simulink model "testCurrentPMSM"  (R2023a)
settings: Solver=ode15s  StartTime=0.0  StopTime=2.0  RelTol=1e-3
libraries: slpidlib x2, eePmsmFieldOrientedControl x1
settings Model: Creator=admin  LastModifiedBy=admin

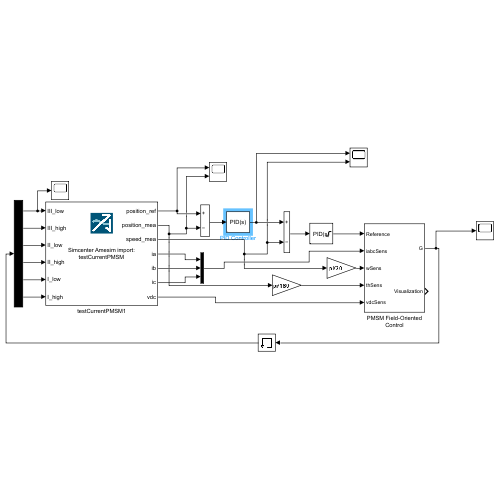
[thumbnail: Simulink's stored preview of the top-level diagram]
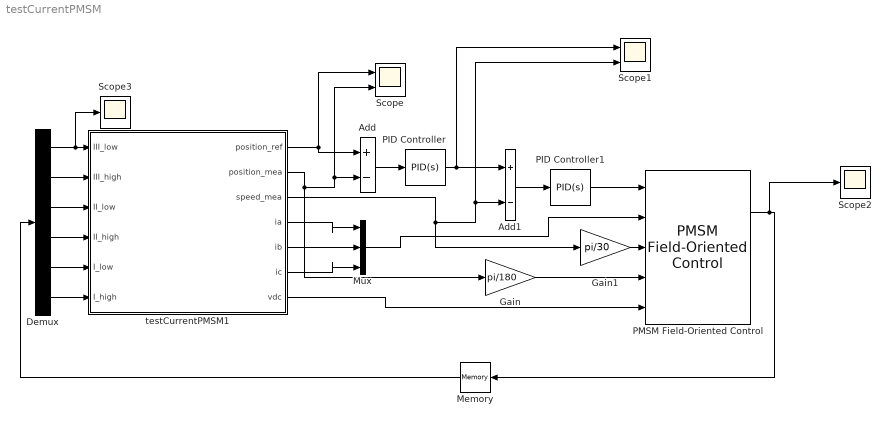
== system testCurrentPMSM ==
  Add : Sum  Inputs=+-
  Add1 : Sum  Inputs=+-
  Demux : Demux  Outputs=6
  Gain : Gain  Gain=pi/180
  Gain1 : Gain  Gain=pi/30
  Memory : Memory
  Mux : Mux  Inputs=3
  PID Controller : slpidlib/PID Controller  Controller=PID  Form=Parallel  TimeDomain=Continuous-time  UseExternalTs=off  SampleTime=-1  IntegratorMethod=Forward Euler  FilterMethod=Forward Euler  ControllerParametersSource=internal  P=1  I=0  UseKiTs=off  D=0  N=100  UseFilter=on  TunerSelectOption=Transfer Function Based (PID Tuner App)  InitialConditionSource=internal  InitialConditionForIntegrator=0  InitialConditionForFilter=0  DifferentiatorICPrevScaledInput=0  ExternalReset=none  TrackingMode=off  Kt=1  LimitOutput=off  SatLimitsSource=internal  UpperSaturationLimit=1000  LowerSaturationLimit=-1000  LinearizeAsGain=on  AntiWindupMode=none  Kb=1  LimitIntegrator=off  UpperIntegratorSaturationLimit=inf  LowerIntegratorSaturationLimit=-inf  POutMin=[]  POutMax=[]  IOutMin=[]  IOutMax=[]  DOutMin=[]  DOutMax=[]  NOutMin=[]  NOutMax=[]  SumOutMin=[]  SumOutMax=[]  SaturationOutMin=[]  SaturationOutMax=[]  PParamMin=[]  PParamMax=[]  IParamMin=[]  IParamMax=[]  DParamMin=[]  DParamMax=[]  NParamMin=[]  NParamMax=[]  KbParamMin=[]  KbParamMax=[]  KtParamMin=[]  KtParamMax=[]  KbOutMin=[]  KbOutMax=[]  KtOutMin=[]  KtOutMax=[]  IntegratorOutMin=[]  IntegratorOutMax=[]  FilterOutMin=[]  FilterOutMax=[]  SumI1OutMin=[]  SumI1OutMax=[]  SumI2OutMin=[]  SumI2OutMax=[]  SumI3OutMin=[]  SumI3OutMax=[]  SumI4OutMin=[]  SumI4OutMax=[]  SumDOutMin=[]  SumDOutMax=[]  DifferentiatorOutMin=[]  DifferentiatorOutMax=[]  FilterDiffOutCoefMin=[]  FilterDiffOutCoefMax=[]  ReciprocalOutMin=[]  ReciprocalOutMax=[]  SumDenOutMin=[]  SumDenOutMax=[]  SumNumOutMin=[]  SumNumOutMax=[]  DivideOutMin=[]  DivideOutMax=[]  UdiffTsProdOutMin=[]  UdiffTsProdOutMax=[]  NTsProdOutMin=[]  NTsProdOutMax=[]  UintegralTsProdOutMin=[]  UintegralTsProdOutMax=[]  UngainTsProdOutMin=[]  UngainTsProdOutMax=[]  ClampingZeroOutDataTypeStr=Inherit: Inherit via back propagation  ClampingZeroOutMin=[]  ClampingZeroOutMax=[]  FilterDenConstantOutDataTypeStr=Inherit: Inherit via back propagation  FilterDenConstantOutMin=[]  FilterDenConstantOutMax=[]  PCopyOutDataTypeStr=Inherit: Inherit via back propagation  PCopyOutMin=[]  PCopyOutMax=[]  NCopyOutDataTypeStr=Inherit: Inherit via back propagation  NCopyOutMin=[]  NCopyOutMax=[]  IntegratorContinuousStateAttributes=''  IntegratorStateMustResolveToSignalObject=off  IntegratorRTWStateStorageClass=Auto  FilterContinuousStateAttributes=''  FilterStateMustResolveToSignalObject=off  FilterRTWStateStorageClass=Auto  ParallelPVariant=InternalParameters  IdealPVariant=Disabled  IVariant=InternalParameters  DVariant=InternalParameters  IntegratorVariant=Continuous  SatVariant=Disabled  AWVariant=Passthrough  PCopyVariant=Disabled  TRVariant=Disabled  FdbkBlocksVariant=Forward  IdealPFdbkVariant=Disabled  SatFdbkVariant=Disabled  DerivativeFilterVariant=ContFilter  NVariant=InternalParameters  NCopyVariant=Disabled  FilterICVariant=InternalICsFilter  IntegratorICVariant=InternalICs  ExternalResetVariant=Disabled  TRSumVariant=Passthrough  SumFdbkVariant=Disabled  SumVariant=Sum_PID  TsampFilterVariant=InternalTs  TsampNgainVariant=Passthrough  TsampIntegralVariant=Disabled_SignalSpec  ExternalSaturationOutDataTypeStr=Inherit: Same as second input
  PID Controller1 : slpidlib/PID Controller  Controller=PID  Form=Parallel  TimeDomain=Continuous-time  UseExternalTs=off  SampleTime=-1  IntegratorMethod=Forward Euler  FilterMethod=Forward Euler  ControllerParametersSource=internal  P=2  I=0.1  UseKiTs=off  D=0  N=100  UseFilter=on  TunerSelectOption=Transfer Function Based (PID Tuner App)  InitialConditionSource=internal  InitialConditionForIntegrator=0  InitialConditionForFilter=0  DifferentiatorICPrevScaledInput=0  ExternalReset=none  TrackingMode=off  Kt=1  LimitOutput=on  SatLimitsSource=internal  UpperSaturationLimit=250  LowerSaturationLimit=-250  LinearizeAsGain=on  AntiWindupMode=none  Kb=1  LimitIntegrator=off  UpperIntegratorSaturationLimit=inf  LowerIntegratorSaturationLimit=-inf  POutMin=[]  POutMax=[]  IOutMin=[]  IOutMax=[]  DOutMin=[]  DOutMax=[]  NOutMin=[]  NOutMax=[]  SumOutMin=[]  SumOutMax=[]  SaturationOutMin=[]  SaturationOutMax=[]  PParamMin=[]  PParamMax=[]  IParamMin=[]  IParamMax=[]  DParamMin=[]  DParamMax=[]  NParamMin=[]  NParamMax=[]  KbParamMin=[]  KbParamMax=[]  KtParamMin=[]  KtParamMax=[]  KbOutMin=[]  KbOutMax=[]  KtOutMin=[]  KtOutMax=[]  IntegratorOutMin=[]  IntegratorOutMax=[]  FilterOutMin=[]  FilterOutMax=[]  SumI1OutMin=[]  SumI1OutMax=[]  SumI2OutMin=[]  SumI2OutMax=[]  SumI3OutMin=[]  SumI3OutMax=[]  SumI4OutMin=[]  SumI4OutMax=[]  SumDOutMin=[]  SumDOutMax=[]  DifferentiatorOutMin=[]  DifferentiatorOutMax=[]  FilterDiffOutCoefMin=[]  FilterDiffOutCoefMax=[]  ReciprocalOutMin=[]  ReciprocalOutMax=[]  SumDenOutMin=[]  SumDenOutMax=[]  SumNumOutMin=[]  SumNumOutMax=[]  DivideOutMin=[]  DivideOutMax=[]  UdiffTsProdOutMin=[]  UdiffTsProdOutMax=[]  NTsProdOutMin=[]  NTsProdOutMax=[]  UintegralTsProdOutMin=[]  UintegralTsProdOutMax=[]  UngainTsProdOutMin=[]  UngainTsProdOutMax=[]  ClampingZeroOutDataTypeStr=Inherit: Inherit via back propagation  ClampingZeroOutMin=[]  ClampingZeroOutMax=[]  FilterDenConstantOutDataTypeStr=Inherit: Inherit via back propagation  FilterDenConstantOutMin=[]  FilterDenConstantOutMax=[]  PCopyOutDataTypeStr=Inherit: Inherit via back propagation  PCopyOutMin=[]  PCopyOutMax=[]  NCopyOutDataTypeStr=Inherit: Inherit via back propagation  NCopyOutMin=[]  NCopyOutMax=[]  IntegratorContinuousStateAttributes=''  IntegratorStateMustResolveToSignalObject=off  IntegratorRTWStateStorageClass=Auto  FilterContinuousStateAttributes=''  FilterStateMustResolveToSignalObject=off  FilterRTWStateStorageClass=Auto  ParallelPVariant=InternalParameters  IdealPVariant=Disabled  IVariant=InternalParameters  DVariant=InternalParameters  IntegratorVariant=Continuous  SatVariant=Enabled  AWVariant=Passthrough  PCopyVariant=Disabled  TRVariant=Disabled  FdbkBlocksVariant=Forward  IdealPFdbkVariant=Disabled  SatFdbkVariant=Disabled  DerivativeFilterVariant=ContFilter  NVariant=InternalParameters  NCopyVariant=Disabled  FilterICVariant=InternalICsFilter  IntegratorICVariant=InternalICs  ExternalResetVariant=Disabled  TRSumVariant=Passthrough  SumFdbkVariant=Disabled  SumVariant=Sum_PID  TsampFilterVariant=InternalTs  TsampNgainVariant=Passthrough  TsampIntegralVariant=Disabled_SignalSpec  ExternalSaturationOutDataTypeStr=Inherit: Same as second input
  PMSM Field-Oriented Control : eePmsmFieldOrientedControl/PMSM Field-Oriented Control  winding_type=Wye-wound  CtrlMode=Torque control  Vnom=450  Pmax=48000  Tmax=440  p=4  Vdc_on=450  Ts=5e-6  Tsc=1e-4  CtrlType=PI control  Kp_w=1  Ki_w=1  Kv_w=1  Kaw_w=1  RefType=Zero d-axis control  rpmVec=[0, 3000]  TqVec=[-100, 0, 100]  VdcVec=[300, 350]  PWMMode=SVM: space vector modulation  ModFactor=1  idMatrix=zeros(2,3,2)  iqMatrix=zeros(2,3,2)  psim=0.0025  Ld=0.00024  Lq=0.00029  Rs=0.01  AxisAlignment=Q-axis  Kp_id=1  Ki_id=2  Kaw_id=1  Kp_iq=1  Ki_iq=2  Kaw_iq=1  AxisPrio=Q-axis  ActZC=off  ActFF=on  ParamTypeFF=Constant parameters  LdFF=0.00024  LqFF=0.00024  psimFF=0.0025  idVect=[-200, 0, 200]  iqVect=[-200, 0, 200]  LdMatrix=0.0002 * ones(3, 3)  LqMatrix=0.0002 * ones(3, 3)  psimMatrix=0.04 * ones(3, 3)  CPWMMode=SVM: space vector modulation  fsw=10000
      settings: LibrarySourceBlock=|
      | ee_sl_lib/PMSM Control/PMSM Field-Oriented
      | Control
  Scope : Scope  NumInputPorts=2
  Scope1 : Scope  NumInputPorts=2
  Scope2 : Scope
  Scope3 : Scope
  testCurrentPMSM1 : Subsystem  Tag=AME2SL  InitFcn=AMESimLib_initBlock  StartFcn=AMESimLib_startBlock  StopFcn=AMESimLib_stopBlock
      settings: DeleteFcn=AMESimLib_deleteBlock  OpenFcn=AMESimLib_openBlock('AME2SL')
      mask Display: image(imread('amesim_pix256.png'),[0.4,0.7,0.2,0.2]);disp('Simcenter Amesim import:\ntestCurrentPMSM');port_label('input',1,'III_low');port_label('input',2,'III_high');port_label('input',3,'II_low');port_label('input',4,'II_high');port_label('input',5,'I_low');port_label('input',6,'I_high');port_label('output',1,'position_ref');port_label('output',2,'position_mea');port_label('output',3,'speed_mea');port_label('output',4,'ia');port_label('output',5,'ib');port_label('output',6,'ic');port_label('output',7,'vdc');
  wires:
  testCurrentPMSM1/1(position_ref) -> Add/1, Scope/1
  Add/1 -> PID Controller/1
  PID Controller/1 -> Add1/1, Scope1/1
  Add1/1 -> PID Controller1/1
  testCurrentPMSM1/2(position_mea) -> Gain/1, Add/2, Scope/2
  testCurrentPMSM1/3(speed_mea) -> Gain1/1, Add1/2, Scope1/2
  PID Controller1/1 -> PMSM Field-Oriented Control/1
  Demux/1 -> Scope3/1, testCurrentPMSM1/1(III_low)
  Demux/2 -> testCurrentPMSM1/2(III_high)
  Demux/3 -> testCurrentPMSM1/3(II_low)
  Demux/4 -> testCurrentPMSM1/4(II_high)
  Demux/5 -> testCurrentPMSM1/5(I_low)
  Demux/6 -> testCurrentPMSM1/6(I_high)
  Gain/1 -> PMSM Field-Oriented Control/4
  Gain1/1 -> PMSM Field-Oriented Control/3
  testCurrentPMSM1/7(vdc) -> PMSM Field-Oriented Control/5
  testCurrentPMSM1/4(ia) -> Mux/1
  testCurrentPMSM1/5(ib) -> Mux/2
  testCurrentPMSM1/6(ic) -> Mux/3
  Mux/1 -> PMSM Field-Oriented Control/2
  PMSM Field-Oriented Control/1 -> Scope2/1, Memory/1
  Memory/1 -> Demux/1

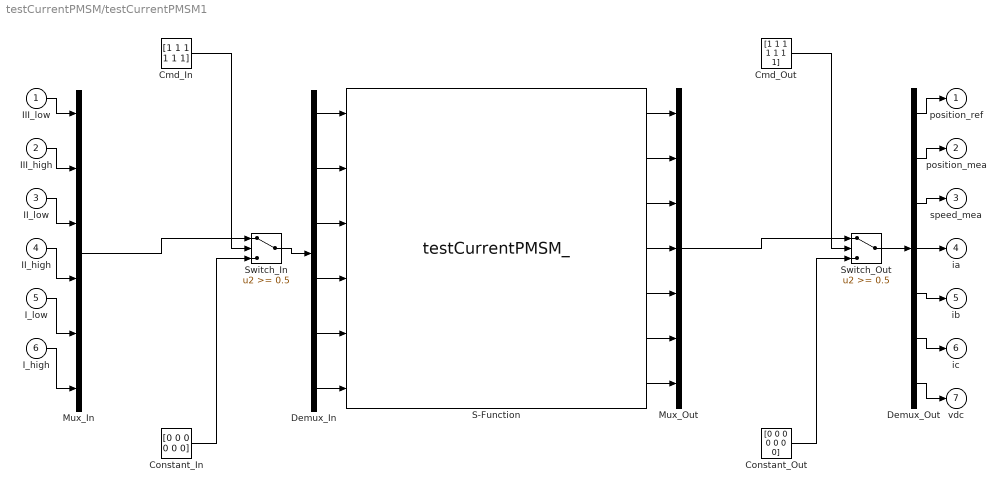
== system testCurrentPMSM/testCurrentPMSM1 ==
  III_low : Inport
  III_high : Inport  Port=2
  II_low : Inport  Port=3
  II_high : Inport  Port=4
  I_low : Inport  Port=5
  I_high : Inport  Port=6
  Cmd_In : Constant  Value=[1 1 1 1 1 1]
  Cmd_Out : Constant  Value=[1 1 1 1 1 1 1]
  Constant_In : Constant  Value=[0 0 0 0 0 0]
  Constant_Out : Constant  Value=[0 0 0 0 0 0 0]
  Demux_In : Demux  Outputs=6
  Demux_Out : Demux  Outputs=7
  Mux_In : Mux  Inputs=6
  Mux_Out : Mux  Inputs=7
  S-Function : S-Function  InitFcn=clear testCurrentPMSM_  StopFcn=clear testCurrentPMSM_  FunctionName=testCurrentPMSM_  Parameters=[1,0.0001] [] [] [] [] [] []  SFunctionDeploymentMode=off  EnableBusSupport=off
      mask Display: port_label('output',1,'position_ref');port_label('output',2,'position_mea');port_label('output',3,'speed_mea');port_label('output',4,'ia');port_label('output',5,'ib');port_label('output',6,'ic');port_label('output',7,'vdc');port_label('input',1,'III_low');port_label('input',2,'III_high');port_label('input',3,'II_low');port_label('input',4,'II_high');port_label('input',5,'I_low');port_label('input',6,'I_high');disp('Simcenter Amesim:\n testCurrentPMSM_')
  Switch_In : Switch  Threshold=0.5
  Switch_Out : Switch  Threshold=0.5
  position_ref : Outport
  position_mea : Outport  Port=2
  speed_mea : Outport  Port=3
  ia : Outport  Port=4
  ib : Outport  Port=5
  ic : Outport  Port=6
  vdc : Outport  Port=7
  wires:
  Mux_In/1 -> Switch_In/1
  Cmd_In/1 -> Switch_In/2
  Constant_In/1 -> Switch_In/3
  Switch_In/1 -> Demux_In/1
  Mux_Out/1 -> Switch_Out/1
  Cmd_Out/1 -> Switch_Out/2
  Constant_Out/1 -> Switch_Out/3
  Switch_Out/1 -> Demux_Out/1
  III_low/1 -> Mux_In/1
  Demux_In/1 -> S-Function/1
  III_high/1 -> Mux_In/2
  Demux_In/2 -> S-Function/2
  II_low/1 -> Mux_In/3
  Demux_In/3 -> S-Function/3
  II_high/1 -> Mux_In/4
  Demux_In/4 -> S-Function/4
  I_low/1 -> Mux_In/5
  Demux_In/5 -> S-Function/5
  I_high/1 -> Mux_In/6
  Demux_In/6 -> S-Function/6
  Demux_Out/1 -> position_ref/1
  S-Function/1 -> Mux_Out/1
  Demux_Out/2 -> position_mea/1
  S-Function/2 -> Mux_Out/2
  Demux_Out/3 -> speed_mea/1
  S-Function/3 -> Mux_Out/3
  Demux_Out/4 -> ia/1
  S-Function/4 -> Mux_Out/4
  Demux_Out/5 -> ib/1
  S-Function/5 -> Mux_Out/5
  Demux_Out/6 -> ic/1
  S-Function/6 -> Mux_Out/6
  Demux_Out/7 -> vdc/1
  S-Function/7 -> Mux_Out/7
